simulink model "InitializationDelay"  (R2016a)
settings: Solver=ode1  StartTime=0.0  StopTime=10.0  FixedStep=h  RelTol=1e-3
undefined symbols (not defined in the file): t0
libraries: simulink x1
settings Model: Creator=ahmad  LastModifiedBy=ahmad

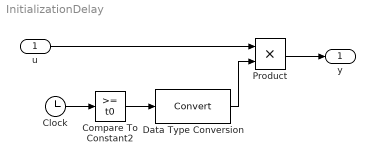
== system InitializationDelay ==
  u : Inport
  Clock : Clock
  Compare To Constant2 : simulink/Logic and Bit Operations/Compare To Constant  relop=>=  const=t0  OutDataTypeStr=boolean
  Data Type Conversion : DataTypeConversion
  Product : Product
  y : Outport
  wires:
  u/1 -> Product/1
  Clock/1 -> Compare To Constant2/1
  Compare To Constant2/1 -> Data Type Conversion/1
  Product/1 -> y/1
  Data Type Conversion/1 -> Product/2
